simulink model "lead_veh_behaviour"  (R2024a)
settings: Solver=VariableStepAuto  StartTime=0  StopTime=1000  RelTol=1e-3
undefined symbols (not defined in the file or in its folder): Defined, Ego, Lane, simStepSize, User
libraries: roadrunnerscenario x3, simulink x2, autolibshared x1
settings Model: Creator=darkh  LastModifiedBy=darkh

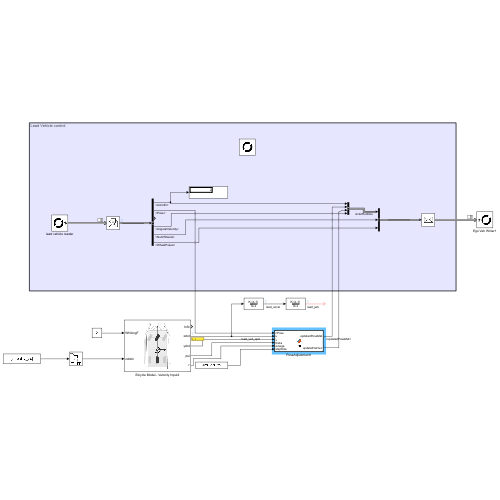
[thumbnail: Simulink's stored preview of the top-level diagram]
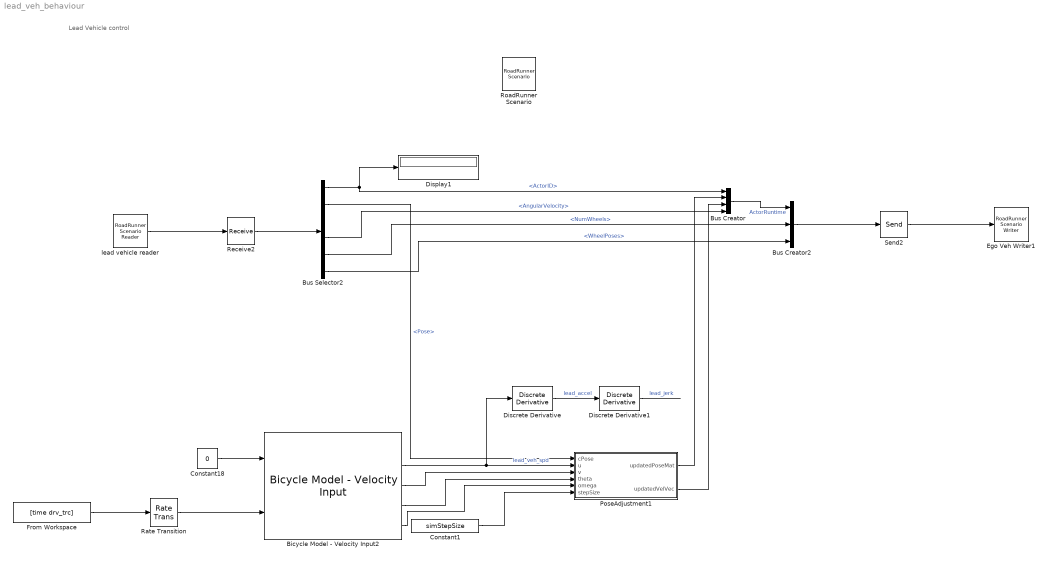
== system lead_veh_behaviour ==
  note: Lead Vehicle control
  Bicycle Model - Velocity Input2 : autolibshared/Bicycle Model - Velocity Input  trackMode=Single (bicycle)  inputMode=External longitudinal velocity  frontSteerMode=on  rearSteerMode=off  windMode=off  muMode=off  extFMode=off  extMMode=off  aMode=3  NF=2  NR=2  m=2630.84  a=1.2  b=1.6  h=0.35  X_o=0  xdot_o=0  CalphaMode=off  sigmaMode=on  w=[1.4,1.4]  Cy_f=19000  Cy_r=33000  sigma_f=.1  sigma_r=.1  alpha_f_brk=[-.1 .1]  Cy_f_data=[-9e3 9e3]  alpha_r_brk=[-.1 .1]  Cy_r_data=[-9e3 9e3]  Y_o=0  ydot_o=0  Izz=2875  psi_o=0  r_o=0  Af=2  Cd=.3  Cl=.1  Cpm=.1  beta_w=[0 0.01:0.01:0.3]  Cs=[0 0.01:0.01:0.3]  Cym=[0 1e-6:0.01:0.3]  Pabs=101325  Tair=273  g=9.81  mu=1  xdot_tol=.01  Fznom=5000  Fxtire_sat=1e6  Fytire_sat=1e6  longOff=0  latOff=0  vertOff=0
      settings: LibrarySourceBlock=drivingscenarioandsensors/Bicycle Model - Velocity Input
  Bus Creator : BusCreator  Inputs=4  OutDataTypeStr=Bus: BusActorRuntime
  Bus Creator2 : BusCreator  Inputs=3  OutDataTypeStr=Bus: BusVehicleRuntime  NonVirtualBus=on
  Bus Selector2 : BusSelector  OutputSignals=ActorRuntime.ActorID,ActorRuntime.Pose,ActorRuntime.Velocity,ActorRuntime.AngularVelocity,NumWheels,WheelPoses
  Constant1 : Constant  Value=simStepSize
  Constant18 : Constant  Value=0
  Discrete Derivative : simulink/Discrete/Discrete Derivative  gainval=1.0  ICPrevScaledInput=0.0  OutMin=[]  OutMax=[]  OutDataType=fixdt(1, 16)  OutScaling=2^-10  DoSatur=off
  Discrete Derivative1 : simulink/Discrete/Discrete Derivative  gainval=1.0  ICPrevScaledInput=0.0  OutMin=[]  OutMax=[]  OutDataType=fixdt(1, 16)  OutScaling=2^-10  DoSatur=off
  Display1 : Display
  Ego Veh Writer1 : roadrunnerscenario/RoadRunner Scenario Writer  TopicCategory=Actor  ActorCategory=Vehicle  EventType=Action Complete  UserDefinedEvent=Event1  VehicleType=Vehicle Pose  TopicType=Actor Pose
  From Workspace : FromWorkspace  VariableName=[time drv_trc]
  PoseAdjustment1 : MATLAB Function  TreatAsAtomicUnit=on
  Rate Transition : RateTransition  OutPortSampleTime=simStepSize
  Receive2 : Receive  InputPortMessageModes=m  UseInternalQueue=off  QueueOverwriting=on  QueueLength=1  QueueType=LIFO
  RoadRunner Scenario : roadrunnerscenario/RoadRunner Scenario  UserDefinedActions={}  UserDefinedEvents={}
  Send2 : Send  OutputPortMessageModes=m
  lead vehicle reader : roadrunnerscenario/RoadRunner Scenario Reader  TopicCategory=Actor  ActorCategory=Vehicle  ActionType=Path Following  EventType=User-Defined  TopicType=Actor Pose  VehicleType=Vehicle Pose  UserDefinedAction=Action1  UserDefinedEvent=Event1  Filter=None  SensorTopic=Target Poses  LaneBoundaryOutputTopic=Ego-Lane  SensorID=1  SampleTime=simStepSize
  wires:
  PoseAdjustment1/1(updatedPoseMat) -> Bus Creator/2
  Bus Creator2/1 -> Send2/1
  Bicycle Model - Velocity Input2/2 -> Discrete Derivative/1, PoseAdjustment1/2(u)  "lead_veh_spd"
  Send2/1 -> Ego Veh Writer1/1
  Bus Selector2/1 -> Bus Creator/1, Display1/1  "<ActorID>"
  Bus Creator/1 -> Bus Creator2/1  "ActorRuntime"
  Bus Selector2/5 -> Bus Creator2/2  "<NumWheels>"
  Bus Selector2/6 -> Bus Creator2/3  "<WheelPoses>"
  Bicycle Model - Velocity Input2/3 -> PoseAdjustment1/3(v)
  Bicycle Model - Velocity Input2/5 -> PoseAdjustment1/5(omega)
  Constant18/1 -> Bicycle Model - Velocity Input2/1
  PoseAdjustment1/2(updatedVelVec) -> Bus Creator/3
  Bus Selector2/2 -> PoseAdjustment1/1(cPose)  "<Pose>"
  lead vehicle reader/1 -> Receive2/1
  Receive2/1 -> Bus Selector2/1
  Bus Selector2/4 -> Bus Creator/4  "<AngularVelocity>"
  Bicycle Model - Velocity Input2/4 -> PoseAdjustment1/4(theta)
  Constant1/1 -> PoseAdjustment1/6(stepSize)
  From Workspace/1 -> Rate Transition/1
  Rate Transition/1 -> Bicycle Model - Velocity Input2/2
  Discrete Derivative/1 -> Discrete Derivative1/1  "lead_accel"
  Discrete Derivative1/1 -> ?  "lead_jerk"

== matlab function lead_veh_behaviour/PoseAdjustment1 ==
  data: cPose input; u input; updatedPoseMat output; v input; theta input; omega input; updatedVelVec output; stepSize input
function [updatedPoseMat, updatedVelVec] = fcn(cPose, u, v, theta, omega, stepSize)
    thetad = theta + omega*stepSize;
    xd = (u*cos(theta) - v*sin(theta))*stepSize;
    yd = (u*sin(theta) + v*cos(theta))*stepSize;
    pose_mat = [cos(-thetad) -sin(-thetad) 0 (yd+cPose(1,4)); sin(-thetad) cos(-thetad) 0 (xd+cPose(2,4)); 0 0 1 0; 0 0 0 1];
    updatedPoseMat = pose_mat;
    updatedVelVec = [u*sin(theta) + v*cos(theta), u*cos(theta) - v*sin(theta), 0];
    return;
end
